simulink model "nav_flocking4"  (R2022b)
settings: Solver=FixedStepAuto  StartTime=0.0  StopTime=10.0  FixedStep=0.01  RelTol=1e-3
values from neighbouring files (symbols this model uses):
  a = 1    [main_flock3.m]    (also in main_flock4.m; params_flocking_ros.m)
  aR = diag([ar; ap; ay])    [main_flock3.m]    (also in main_flock4.m; main_sliding.m)
  Att1 = [2 -2 -15]    [main_flock3.m]    (also in main_flock4.m)
  Att2 = [2 -2 -15]    [main_flock3.m]    (also in main_flock4.m)
  Att3 = [2 -2 -15]    [main_flock3.m]    (also in main_flock4.m)
  Att4 = [2 -2 -15]    [main_flock4.m]
  b = 1    [main_flock3.m]    (also in main_flock4.m; params_flocking_ros.m)
  c = 1    [main_flock3.m]    (also in main_flock4.m; params_flocking_ros.m)
  c_gammap = 1.2    [main_flock3.m]    (also in main_flock4.m)
  c_gammav = 3.5    [main_flock3.m]    (also in main_flock4.m)
  d = 0.6    [main_flock3.m]    (also in main_flock4.m; params_flocking_ros.m)
  d_prime = 1    [main_flock3.m]    (also in main_flock4.m; params_flocking_ros.m)
  epsilon = 0.1    [main_flock3.m]    (also in main_flock4.m; params_flocking_ros.m)
  h = 0.2    [main_flock3.m]    (also in main_flock4.m; params_flocking_ros.m)
  K1 = diag([k111; k122; k133])    [main_flock3.m]    (also in main_flock4.m; main_sliding.m)
  K2 = diag([k211; k222; k233])    [main_flock3.m]    (also in main_flock4.m; main_sliding.m)
  Ki = diag([Ki1; Ki2; Ki3])    [main_flock3.m]    (also in main_flock4.m; main_sliding.m)
  lam = diag([lam1; lam2; lam3])    [main_flock3.m]    (also in main_flock4.m; main_sliding.m)
  R = 0.15    [main_flock3.m]    (also in main_flock4.m; params_flocking_ros.m)
  vxobs = 0    [main_flock3.m]    (also in main_flock4.m)
  vyobs = 0    [main_flock3.m]    (also in main_flock4.m)
  vzobs = 0    [main_flock3.m]    (also in main_flock4.m)
  X0_1 = [P01 dP01 om01]    [main_flock3.m]    (also in main_flock4.m; main_sliding.m = [P0 dP0 om0])
  X0_2 = [P02 dP02 om02]    [main_flock3.m]    (also in main_flock4.m)
  X0_3 = [P03 dP03 om03]    [main_flock3.m]    (also in main_flock4.m)
  X0_4 = [P04 dP04 om04]    [main_flock4.m]
  xmax = 2    [main_flock3.m]    (also in main_flock4.m)
  xmin = -2    [main_flock3.m]    (also in main_flock4.m)
  xobs = 0.75    [main_flock3.m]    (also in main_flock4.m)
  yobs = -0.25    [main_flock3.m]    (also in main_flock4.m)
  zobs = 1.7    [main_flock3.m]    (also in main_flock4.m)
undefined symbols (not defined in the file or in its folder): A_Euler
libraries: aerosimlib x4
(part 3 of 3)

== matlab function nav_flocking4/Translational Control4/Flocking1/MATLAB Function1 ==
  data: phiAlpha input; phiAlpha_int input; aie input; aive input; ui_gamma input; phiBetak input; bikobs input; phiBetanei input; bikve input; Ui output size=3; KP parameter

function Ui  = ctrlLaw(phiAlpha, phiAlpha_int, aie, aive, ui_gamma, phiBetak, bikobs, phiBetanei, bikve, KP)  %, phiBetak, phiBetanei
    
    % Control gains and parameters
    Kx = KP(1); Ky = KP(2); Kz = KP(3);
    Kpx = KP(4); Kpy = KP(5); Kpz = KP(6);
    Kdx = KP(7); Kdy = KP(8); Kdz = KP(9);
    Kix = KP(10); Kiy = KP(11); Kiz = KP(12);
    cBetax = KP(13); cBetay = KP(14); cBetaz = KP(15);
    cdBetax = KP(16); cdBetay = KP(17); cdBetaz = KP(18);
    
        
    hx_dot = Kx * phiAlpha(1,1) + Kpx * aie(1,1) + Kdx * aive(1,1) + Kix * phiAlpha_int(1,1) + ui_gamma(1,1) + cBetax * (phiBetak(1,1) + phiBetanei(1,1)) + cdBetax * (bikobs(1,1) + bikve(1,1));
    hy_dot = Ky * phiAlpha(2,1) + Kpy * aie(2,1) + Kdy * aive(2,1) + Kiy * phiAlpha_int(2,1) + ui_gamma(2,1) + cBetay * (phiBetak(2,1) + phiBetanei(2,1)) + cdBetay * (bikobs(2,1) + bikve(2,1));
    hz_dot = Kz * phiAlpha(3,1) + Kpz * aie(3,1) + Kdz * aive(3,1) + Kiz * phiAlpha_int(3,1) + ui_gamma(3,1) + cBetaz * (phiBetak(3,1) + phiBetanei(3,1)) + cdBetaz * (bikobs(3,1) + bikve(3,1));
    

    Ui = [hx_dot; hy_dot; hz_dot] ;
        
end

== matlab function nav_flocking4/Translational Control4/Flocking1/MATLAB Function2 ==
  data: xi input; yi input; zi input; vxi input; vyi input; vzi input; ui_gamma output; xr input; yr input; zr input; vxr input; vyr input; vzr input; c_gammap parameter; xmin parameter; xmax parameter; c_gammav parameter

function ui_gamma   = naviFeedback(xi, yi, zi, vxi, vyi, vzi, xr, yr, zr, vxr, vyr, vzr, c_gammap, xmin, xmax, c_gammav)
    
       
    Pi = [xi ; yi ; zi] ;
    Vi = [vxi ; vyi ; vzi] ;


    Pr = [xr ; yr ; zr] ;
    Vr = [vxr ; vyr ; vzr] ;
    
    ui_gamma = (-1).* satFcn(c_gammap.*(Pi - Pr), xmin, xmax) + (-1).* satFcn(c_gammav.*(Vi - Vr), xmin, xmax) ;
    
end

== matlab function nav_flocking4/Translational Control4/Flocking1/MATLAB Function3 ==
  data: xi input; yi input; zi input; vxi input; vyi input; vzi input; xobs parameter; yobs parameter; zobs parameter; vxobs parameter; vyobs parameter; vzobs parameter; phiBetanik output; R parameter; epsilon parameter; d_prime parameter; h parameter; bikobs output
function [phiBetanik, bikobs] = phiBetaFcn(xi, yi, zi, vxi, vyi, vzi, xobs, yobs, zobs, vxobs, vyobs, vzobs, R, epsilon, d_prime, h)
    
    dBeta = sigmaNormFun(d_prime, epsilon) ;
    
    Pi = [xi ; yi ; zi] ;
    Pc = [xobs ; yobs ; zobs] ;
    
    Vi = [vxi ; vyi ; vzi] ;
    Vc = [vxobs ; vyobs ; vzobs] ;

    % Compute closest point between the robot center and the obstacle
    % circumference (ossumming obstacles are circles)
    Pk = Pc + (Pi - Pc) * (R /norm(Pi - Pc)) ;
    %Pk = [xobs ; yobs] ;
    
    sigmaNormk = sigmaNormFun(Pk - Pi, epsilon) ;
    nik = gradSigmaFun(Pk - Pi, epsilon) ;
    
    sigma1k = sigma1Fun(sigmaNormk - dBeta) ;
    
    %% Position
    phiBetak = bumpFcn(sigmaNormk/dBeta,h) * (sigma1k - 1) ;
    phiBetanik = phiBetak.* nik ;
    
    %% Velocity
    bikobs = bumpFcn(sigmaNormk/dBeta,h).*(Vc + (Vi - Vc));
end

== matlab function nav_flocking4/Translational Control4/Flocking1/MATLAB Function4 ==
  data: xj input; yj input; zj input; vxj input; vyj input; vzj input; xk input; yk input; zk input; vxk input; vyk input; vzk input; xl input; yl input; zl input; vxl input; vyl input; vzl input; xobs parameter; yobs parameter; zobs parameter; phiBetaniknei output; R parameter; epsilon parameter; d_prime parameter; h parameter; vxobs parameter; vyobs parameter; vzobs parameter; bikve output
function [phiBetaniknei, bikve] = phiBetaFcn(xj, yj, zj, vxj, vyj, vzj, xk, yk, zk, vxk, vyk, vzk, xl, yl, zl, vxl, vyl, vzl, xobs, yobs, zobs, R, epsilon, d_prime, h, vxobs, vyobs, vzobs)
    
    dBeta = sigmaNormFun(d_prime, epsilon) ;
    
    Pj = [xj ; yj ; zj] ;
    Pk = [xk ; yk ; zk] ;
    Pl = [xl ; yl ; zl] ;
    Pc = [xobs ; yobs ; zobs] ;

    Vj = [vxj ; vyj ; vzj] ;
    Vk = [vxk ; vyk ; vzk] ;
    Vl = [vxl ; vyl ; vzl] ;
    Vc = [vxobs ; vyobs ; vzobs] ;

    % Compute closest point between the robot center and the obstacle
    % circumference (ossumming obstacles are circles)
    Pobsj = Pc + (Pj - Pc) * (R /norm(Pj - Pc)) ;
    Pobsk = Pc + (Pk - Pc) * (R /norm(Pk - Pc)) ;
    Pobsl = Pc + (Pl - Pc) * (R /norm(Pl - Pc)) ;
    %Pk = [xobs ; yobs] ;
    
    %%
    sigmaNormj = sigmaNormFun(Pobsj - Pj, epsilon) ;
    nij = gradSigmaFun(Pobsj - Pj, epsilon) ;
    
    sigmaNormk = sigmaNormFun(Pobsk - Pk, epsilon) ;
    nik = gradSigmaFun(Pobsk - Pk, epsilon) ;

    sigmaNorml = sigmaNormFun(Pobsl - Pl, epsilon) ;
    nil = gradSigmaFun(Pobsl - Pl, epsilon) ;

    %%
    sigma1j = sigma1Fun(sigmaNormj - dBeta) ;
    sigma1k = sigma1Fun(sigmaNormk - dBeta) ;
    sigma1l = sigma1Fun(sigmaNorml - dBeta) ;
            
    %%
    phiBetaj = bumpFcn(sigmaNormj/dBeta,h) * (sigma1j - 1) ;
    phiBetak = bumpFcn(sigmaNormk/dBeta,h) * (sigma1k - 1) ;
    phiBetal = bumpFcn(sigmaNorml/dBeta,h) * (sigma1l - 1) ;
            
    %% Position
    phiBetaniknei = phiBetaj.* nij + phiBetak.* nik + phiBetal.* nil;
    
    %% Velocity
    bikve = bumpFcn(sigmaNormj/dBeta,h).*(Vc + (Vj - Vc)) + bumpFcn(sigmaNormk/dBeta,h).*(Vc + (Vk - Vc)) + bumpFcn(sigmaNorml/dBeta,h).*(Vc + (Vl - Vc));
end

== matlab function nav_flocking4/Translational Control4/to_desired_angles ==
  data: Gamma input; cq_d output; Uz output
function [cq_d,Uz] = fcn(Gamma)

%Physical parameters
m = 0.65;
g = 9.81;

%Control signals separation
gamma = Gamma(1:3);
gamma1 = gamma(1);
gamma2 = gamma(2);
gamma3 = gamma(3);

%Desired Phi, theta, trust
psi = 0*pi/180;

phi = atan(gamma2/(gamma3+g));

theta = asin(-gamma1/(sqrt(gamma1^2+gamma2^2+(gamma3+g)^2)));

Uz = m*sqrt((gamma1)^2+(gamma2)^2+(gamma3+g)^2);

%Conversion to quaternions
q0 = cos(psi/2)*cos(theta/2)*cos(phi/2) + sin(psi/2)*sin(theta/2)*sin(phi/2);
q1 = cos(psi/2)*cos(theta/2)*sin(phi/2) - sin(psi/2)*sin(theta/2)*cos(phi/2);
q2 = cos(psi/2)*sin(theta/2)*cos(phi/2) + sin(psi/2)*cos(theta/2)*sin(phi/2);
q3 = sin(psi/2)*cos(theta/2)*cos(phi/2) - cos(psi/2)*sin(theta/2)*sin(phi/2);

cq_d = [q0;
        -q1;
        -q2;
        -q3];

== matlab function nav_flocking4/Dron_dynamics/Mixer (Parrot ARDRONE) ==
  data: T input; w1 output size=1; tau input; w2 output size=1; w3 output size=1; w4 output size=1
function [w1,w2,w3,w4]   = fcn(T, tau)
%#codegen
tau_phi = tau(1); 
tau_the = tau(2); 
tau_psi = tau(3);

% This values vary in fonction of the geometry of the drone 
b= 4.06e-6;
d= 7.5e-7;
l= (0.2)*(sin(pi/4));

%Parrot AR-DRONE 
uT = T/b; 
uphi = (sqrt(2)*tau_phi)/(b*l);  
uthe = (sqrt(2)*tau_the)/(b*l);
upsi = tau_psi/(d*l);

%Mix by Motors
mixM1 = uT+uphi-uthe+upsi;  %uT + for all mixM
mixM2 = uT-uphi-uthe-upsi; 
mixM3 = uT-uphi+uthe+upsi; 
mixM4 = uT+uphi+uthe-upsi;

%rotors speeds [rads/s]
w1= sign(mixM1)*sqrt(abs((1/4)*mixM1));
w2= sign(mixM2)*sqrt(abs((1/4)*mixM2));
w3= sign(mixM3)*sqrt(abs((1/4)*mixM3));
w4= sign(mixM4)*sqrt(abs((1/4)*mixM4));
